simulink library "aeroutilslib"  (Simulink 6.6)
undefined symbols (not defined in the file or in its folder): DiscIntNeverNeededParam, POS_hi, POS_lo, Timestep
libraries: simulink x13, aeroutilslib x1
settings Model: Creator=cox  LastModifiedBy=la1032aw  ExtModeAutoUpdateStatusClock=off

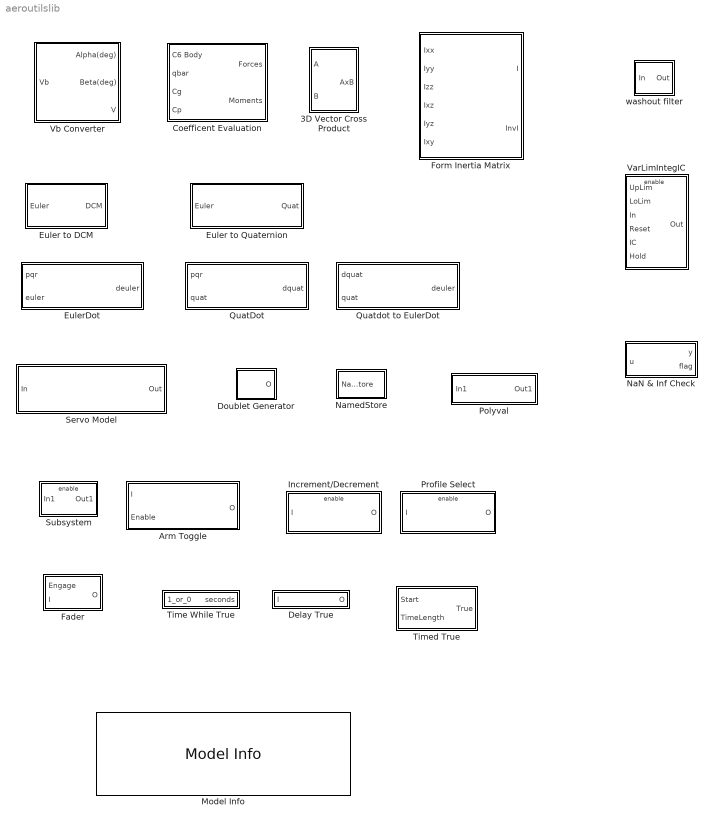
== system aeroutilslib ==
  3D Vector Cross Product : Subsystem
  Arm Toggle : Subsystem
  Coefficent Evaluation : Subsystem  mask{b=1, cbar=1, Sref=1}
      mask prompts: b "Reference Span (b)"; cbar "Reference Chord (cbar)"; Sref "Reference Area (Sref)"
      mask help:
      | Calulates the Force and Moments due to aerodynamic loads from vector of body axes aerodynamic coefficients:
      |    C6body = [Cx Cy Cz Cl Cm Cn].
      | Also requires dynamic pressure, cg/cp locations and reference lengths/area.
  Delay True : Subsystem  mask{holdoff=0, timestep=Timestep}
      mask help: Delays output of "True" value for given time. Outputs boolean. Uses a 32-bit counter instead of a clock source so the output is discrete.
      mask Display: disp([num2str(holdoff) ' sec'])
  Doublet Generator : Subsystem  mask(DoubletGenerator){timeon=[3 10 17], pulsewidth=[2 2 2], amplitude=[0 0 0]}
      mask prompts: timeon "Time Start"; pulsewidth "Pulse Duration"
      mask help:
      | Doublet Generator.
      | Ouputs doublet of specificed amplitude and duration.
      |
      | If start/duration/amplitude parameters are vectors, then output is multichannel.
      mask Display: plot([.1 .3 .3001 .4 .4001 .5  .5001 .7],[0 0 1 1 -1 -1 0 0])
  Euler to DCM : Subsystem
  Euler to Quaternion : Subsystem
  EulerDot : Stateflow chart
  Fader : Subsystem
  Form Inertia Matrix : Stateflow chart
  Increment/Decrement : Subsystem  mask(Increment/Decrement ){Threshold=9}
      mask help:
      | Input is a discrete toggle: +/-1 increments up/down, zero is no change
      | Set the Threshold where the output should wrap around. (1 is the lower limit)
      | Initial value is 1. Output is uint32.
      mask Display: disp(['Threshold: ' num2str(Threshold)])
  Model Info : simulink/Model-Wide Utilities/Model Info  SystemSampleTime=-1  InitialBlockCM=none  BlockCM=none  Frame=on  DisplayStringWithTags=|  HorizontalTextAlignment=Center  LeftAlignmentValue=0.5  SourceBlockDiagram=aeroutilslib  TagMaxNumber=20
      | Aero Utility Library
      | %<ModelVersion>
      | Las modified by %<LastModifiedBy> on %<LastModificationDate>
  NaN & Inf Check : Stateflow chart
  NamedStore : Subsystem  StopFcn=|  mask(Custom To Workspace Block){Npts=inf, VarName=sout, expand=off}
      | %                                                                                       
      | % script: namedstore_stopfcn                                                            
      | %                                                                                       
      | % Workspace script called by NamedStore block as StopFcn callback.                      
      | %                                                                                       
      | % This converts from fixed name array and  variable list                                
      | % into user names structure.   It also optionally expands fields of the                 
      | % structure  into individual variables.                                                 
      |                                                                                         
      | VarName=get_param(gcb,'VarName');                                                       
      |                                                                                         
      |                                                                                         
      | % If data exists                                                                        
      | if exist(strcat(VarName,'_mat'),'var');                                                 
      |   % Grab field names from diagram                                                       
      |    signal_names=get_param(sprintf('%s/Names',gcb),'InputSignals');                      
      |                                                                                         
      |   % Only works for scalar signals...                                                    
      |   % Doing vectors would require pre-compile of diagram,                                 
      |   % and parsing of "CompliedPortDimensions" parameter.                                  
      |   if length(signal_names) ~=  eval(sprintf('size(%s_mat,2)',VarName));                  
      |     fprintf(1,'Structure ''%s'' not formed, namedsore data remains in matrix form\n',...
      |             VarName);                                                                   
      |     error('NamedStore input contains non-scalar signals');                              
      |   end                                                                                   
      |                                                                                         
      |   % Don't want to augment existing variable                                             
      |   eval(sprintf('clear %s',VarName));                                                    
      |                                                                                         
      |   % Loop through each named variable, assign in structure;                              
      |   for cnt=[1:length(signal_names)],                                                     
      |     eval(sprintf('%s.(signal_names{cnt})=%s_mat(:,cnt);',...                            
      |                  VarName,VarName));                                                     
      |   end                                                                                   
      |                                                                                         
      |                                                                                         
      |                                                                                         
      |   % If selected, expand all fields.                                                     
      |   if (strcmp(get_param(gcb,'expand'),'on' ))                                            
      |     eval(sprintf('expand(%s);',VarName));                                               
      |   end                                                                                   
      |  % Delete tmp name variables from workspace                                             
      |   eval(sprintf('clear %s_mat',VarName));                                                
      |   clear cnt VarName signal_names                                                        
      |  end
      mask prompts: Npts "Limit data points to last"; VarName "Variable Name"; expand "Expand Variables in Base Workspace"
      mask help:
      | Saves simulation data to a workspace variable in a structure format.
      | Input is limited to uniquely named scalar signals.
      | Relies on a stop-fcn callback.
      mask init:
      | set_param(sprintf('%s/To Workspace',gcb),'MaxDataPoints',sprintf('%d',Npts));
      | InSig=get_param(sprintf('%s/Names',gcb),'InputSignals');
      | set_param(sprintf('%s/Names',gcb),'OutputSignals',InSig{1});  % Gotta have one..
      | set_param(sprintf('%s/To Workspace',gcb),'VariableName',strcat(VarName,'_mat'));
      | 
      | 
      | 
      | % Check for duplicates, error out
      | [uni,ndx]=unique(InSig);
      | if length(uni)~=length(InSig),
      |  dups=InSig(setdiff([1:length(InSig)],ndx));
      |  dups
      |  error(sprintf('\nDuplicate signal names in named_store block: %s',dups{:}));
      | end
      mask Display: port_label('input',1,VarName);
  Polyval : Subsystem  mask{p=[2 1]}
      mask prompts: p "Polynomial"
      mask help:
      | Embedded MATLAB version of the polyval block.
      | Input polynomial coefficients as a vector in descending order.
      mask Display:
      | disp('y = P(u)\n')
      | disp(['\nO(P) = ' num2str(length(p)-1)])
  Profile Select : Subsystem  mask(Select profile){Profiles=9}
      mask help: Analog input should be normalized between 0 and +1. Block outputs a round number between 1 and the max number of profiles. Output is uint32.
      mask Display: disp(['Profiles: ' num2str(Profiles)])
  QuatDot : Stateflow chart
  Quatdot to EulerDot : Stateflow chart
  Servo Model : Subsystem  mask(Rate and Position Limited Servo){freq=10, RL=999.0, POS_hi=20.0, POS_lo=-30.0}
      mask prompts: freq "Bandwidth, Hz"; RL "Rate Limit:"; POS_hi "Position Limit High:"; POS_lo "Position Limit Low:"
      mask help: First order transfer function: w/(s+w), with rate and position limits.
      mask Help:
      | This block models a first order servo with the initial condition
      | on the integrator set to the steady state value for constant input.
      | The servo is rate and position limited and those values are set
      | in the block parameters.
      mask Display:
      | text(.48,.55,sprintf('%3.1f Hz\nBW',freq),'horizontalAlignment','center');
      | 
      | text(0.18,0.45,sprintf('|d/dt|\n<%0.1f',RL),'horizontalAlignment','center');
      | 
      | text(0.88,0.85,num2str(POS_hi),'horizontalAlignment', 'center');
      | text(0.88,0.2,num2str(POS_lo),'horizontalAlignment', 'center');
      | text(0.73,0.5,'P\nL');
      | 
      | 
      | plot([0.83 0.87 0.93 0.97],[0.4 0.4 0.6 0.6]);
      | plot([0.81 0.99],[0.5 0.5]);
      | plot([0.9 0.9],[0.3 0.7]);
      | plot([0.81 0.99 0.99 0.81 0.81],[0.3 0.3 0.7 0.7 0.3]);
  Subsystem : Subsystem
      mask Type: Toggle Switch
      mask Description: Boolean output toggles between 0 and 1 when an increase is detected in the input
      mask Display: disp('Toggle')
  Time While True : Subsystem  mask{timestep=Timestep}
      mask help: uses a 32-bit and the Timestep variable to output Time While the input signal is true. Output signal is discrete.
  Timed True : Subsystem  mask{timestep=Timestep}
      mask help: Uses a 32-bit counter and the Timestep variable to output a variable time length true signal. Output signal is discrete.
  VarLimIntegIC : Subsystem
  Vb Converter : Subsystem
  washout filter : Subsystem  mask(first order filter){A=1, B=1, C=1}
      mask help:
      | __As__
      |  Bs+C
      |
      | Washout filter  transfer function
      | with integrator IC = input* A/C  at time=0
      mask Help:
      | This block models a washout filter with the initial condition
      | on the integrator set to the steady state value for constant input.
      | A, B and C values are the filter coefficients
      | As / (Bs+C)
      mask Display: dpoly([A 0],[B C]);

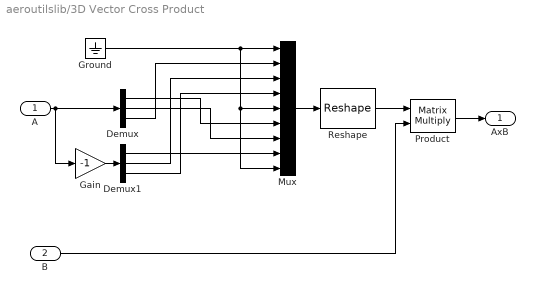
== system aeroutilslib/3D Vector Cross Product ==
  A : Inport
  B : Inport  Port=2
  Demux : Demux  Outputs=3
  Demux1 : Demux  Outputs=3
  Gain : Gain  Gain=-1  SaturateOnIntegerOverflow=on
  Ground : Ground
  Mux : Mux  Inputs=9
  Product : Product  Multiplication=Matrix(*)  SaturateOnIntegerOverflow=on
  Reshape : Reshape  OutputDimensionality=Customize  OutputDimensions=[3,3]
  AxB : Outport
  wires:
  A/1 -> Demux/1, Gain/1
  Product/1 -> AxB/1
  Ground/1 -> Mux/1, Mux/5, Mux/9
  Gain/1 -> Demux1/1
  Demux/3 -> Mux/2
  Demux1/2 -> Mux/3
  Demux1/3 -> Mux/4
  Demux/1 -> Mux/6
  Demux/2 -> Mux/7
  Demux1/1 -> Mux/8
  Mux/1 -> Reshape/1
  Reshape/1 -> Product/1
  B/1 -> Product/2

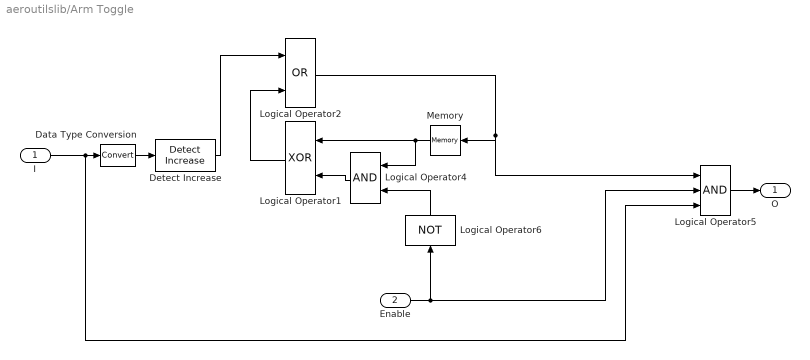
== system aeroutilslib/Arm Toggle ==
  I : Inport
  Enable : Inport  Port=2
  Data Type Conversion : DataTypeConversion  OutDataTypeMode=double
  Detect Increase : simulink/Logic and Bit Operations/Detect Increase  SystemSampleTime=-1  vinit=0.0
  Logical Operator1 : Logic  Orientation=left  Operator=XOR  AllPortsSameDT=off  OutDataTypeMode=Boolean
  Logical Operator2 : Logic  Operator=OR  AllPortsSameDT=off  OutDataTypeMode=Boolean
  Logical Operator4 : Logic  Orientation=left  AllPortsSameDT=off  OutDataTypeMode=Boolean
  Logical Operator5 : Logic  Inputs=3  AllPortsSameDT=off  OutDataTypeMode=Boolean
  Logical Operator6 : Logic  Orientation=up  Operator=NOT  Inputs=3  AllPortsSameDT=off  OutDataTypeMode=Boolean
  Memory : Memory  Orientation=left
  O : Outport
  wires:
  Enable/1 -> Logical Operator6/1, Logical Operator5/2
  Logical Operator2/1 -> Memory/1, Logical Operator5/1
  I/1 -> Logical Operator5/3, Data Type Conversion/1
  Memory/1 -> Logical Operator1/1, Logical Operator4/1
  Logical Operator1/1 -> Logical Operator2/2
  Logical Operator4/1 -> Logical Operator1/2
  Detect Increase/1 -> Logical Operator2/1
  Logical Operator6/1 -> Logical Operator4/2
  Logical Operator5/1 -> O/1
  Data Type Conversion/1 -> Detect Increase/1

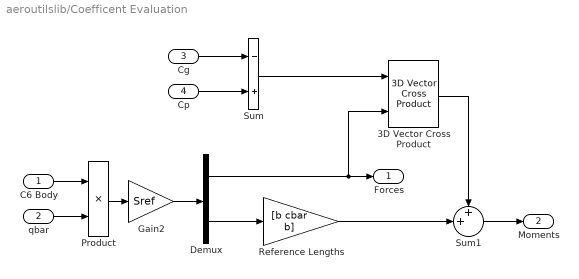
== system aeroutilslib/Coefficent Evaluation ==
  C6 Body : Inport
  qbar : Inport  Port=2
  Cg : Inport  Port=3
  Cp : Inport  Port=4
  3D Vector Cross Product : aeroutilslib/3D Vector Cross Product  SystemSampleTime=-1
  Demux : Demux  Outputs=[3 3]
  Gain2 : Gain  Gain=Sref  SaturateOnIntegerOverflow=on
  Product : Product  SaturateOnIntegerOverflow=on  InputSameDT=on
  Reference Lengths : Gain  Gain=[b cbar b]  SaturateOnIntegerOverflow=on
  Sum : Sum  Inputs=-+  SaturateOnIntegerOverflow=on
  Sum1 : Sum  Inputs=++|  SaturateOnIntegerOverflow=on
  Forces : Outport
  Moments : Outport  Port=2
  wires:
  3D Vector Cross Product/1 -> Sum1/1
  Sum1/1 -> Moments/1
  Reference Lengths/1 -> Sum1/2
  Demux/1 -> Forces/1, 3D Vector Cross Product/2
  Demux/2 -> Reference Lengths/1
  Gain2/1 -> Demux/1
  Product/1 -> Gain2/1
  qbar/1 -> Product/2
  C6 Body/1 -> Product/1
  Cp/1 -> Sum/2
  Cg/1 -> Sum/1
  Sum/1 -> 3D Vector Cross Product/1

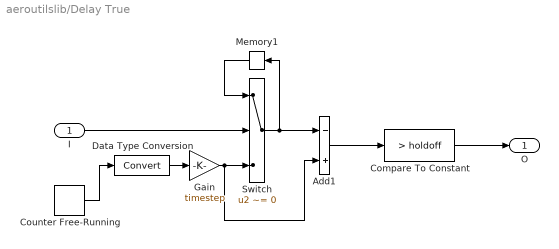
== system aeroutilslib/Delay True ==
  I : Inport
  Add1 : Sum  Inputs=-+  OutScaling=2^-10
  Compare To Constant : simulink/Logic and Bit Operations/Compare To Constant  SystemSampleTime=-1  relop=>  const=holdoff  LogicOutDataTypeMode=boolean  ZeroCross=off
  Counter Free-Running : simulink/Sources/Counter Free-Running  SystemSampleTime=-1  NumBits=32  tsamp=-1
  Data Type Conversion : DataTypeConversion  OutDataTypeMode=double
  Gain : Gain  Gain=timestep
  Memory1 : Memory  Orientation=left
  Switch : Switch  Criteria=u2 ~= 0
  O : Outport
  wires:
  Gain/1 -> Switch/3, Add1/2
  Data Type Conversion/1 -> Gain/1
  Counter Free-Running/1 -> Data Type Conversion/1
  Memory1/1 -> Switch/1
  Switch/1 -> Add1/1, Memory1/1
  I/1 -> Switch/2
  Add1/1 -> Compare To Constant/1
  Compare To Constant/1 -> O/1

== system aeroutilslib/Doublet Generator ==
  Add : Sum  Inputs=+++  OutScaling=2^-10
  DownStep : Step  Time=timeon+pulsewidth  After=-2  SampleTime=0
  Gain : Gain  Gain=amplitude
  UnStep : Step  Time=timeon+2*pulsewidth  SampleTime=0
  UpStep : Step  Time=timeon  SampleTime=0
  O : Outport
  wires:
  UpStep/1 -> Add/1
  DownStep/1 -> Add/2
  UnStep/1 -> Add/3
  Add/1 -> Gain/1
  Gain/1 -> O/1

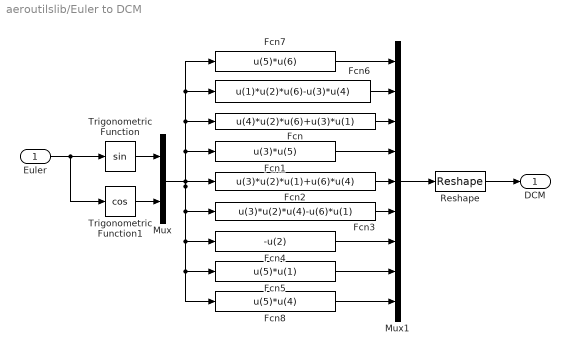
== system aeroutilslib/Euler to DCM ==
  "Euler " : Inport
  Fcn : Fcn  Expr=u(4)*u(2)*u(6)+u(3)*u(1)
  Fcn1 : Fcn  Expr=u(3)*u(5)
  Fcn2 : Fcn  Expr=u(3)*u(2)*u(1)+u(6)*u(4)
  Fcn3 : Fcn  Expr=u(3)*u(2)*u(4)-u(6)*u(1)
  Fcn4 : Fcn  Expr=-u(2)
  Fcn5 : Fcn  Expr=u(5)*u(1)
  Fcn6 : Fcn  Expr=u(1)*u(2)*u(6)-u(3)*u(4)
  Fcn7 : Fcn  Expr=u(5)*u(6)
  Fcn8 : Fcn  Expr=u(5)*u(4)
  Mux : Mux  Inputs=2
  Mux1 : Mux  Inputs=9
  Reshape : Reshape  OutputDimensionality=Customize  OutputDimensions=[3,3]
  Trigonometric Function : Trigonometry
  Trigonometric Function1 : Trigonometry  Operator=cos
  DCM : Outport
  wires:
  "Euler "/1 -> Trigonometric Function1/1, Trigonometric Function/1
  Trigonometric Function/1 -> Mux/1
  Trigonometric Function1/1 -> Mux/2
  Mux/1 -> Fcn/1, Fcn7/1, Fcn6/1, Fcn1/1, Fcn2/1, Fcn4/1, Fcn8/1, Fcn5/1, Fcn3/1
  Mux1/1 -> Reshape/1
  Fcn7/1 -> Mux1/1
  Fcn6/1 -> Mux1/2
  Fcn/1 -> Mux1/3
  Fcn1/1 -> Mux1/4
  Fcn2/1 -> Mux1/5
  Fcn3/1 -> Mux1/6
  Fcn4/1 -> Mux1/7
  Fcn5/1 -> Mux1/8
  Fcn8/1 -> Mux1/9
  Reshape/1 -> DCM/1

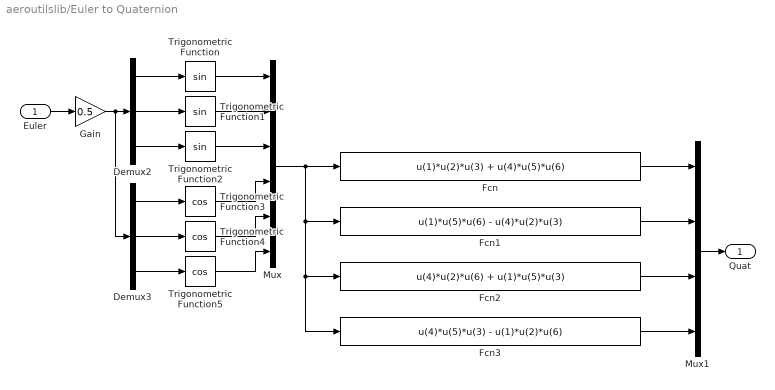
== system aeroutilslib/Euler to Quaternion ==
  Euler : Inport
  Demux2 : Demux  Outputs=3
  Demux3 : Demux  Outputs=3
  Fcn : Fcn  Expr=u(1)*u(2)*u(3) + u(4)*u(5)*u(6)
  Fcn1 : Fcn  Expr=u(1)*u(5)*u(6) - u(4)*u(2)*u(3)
  Fcn2 : Fcn  Expr=u(4)*u(2)*u(6) + u(1)*u(5)*u(3)
  Fcn3 : Fcn  Expr=u(4)*u(5)*u(3) - u(1)*u(2)*u(6)
  Gain : Gain  Gain=0.5
  Mux : Mux  Inputs=6
  Mux1 : Mux
  Trigonometric Function : Trigonometry
  Trigonometric Function1 : Trigonometry
  Trigonometric Function2 : Trigonometry
  Trigonometric Function3 : Trigonometry  Operator=cos
  Trigonometric Function4 : Trigonometry  Operator=cos
  Trigonometric Function5 : Trigonometry  Operator=cos
  Quat : Outport
  wires:
  Gain/1 -> Demux2/1, Demux3/1
  Demux2/1 -> Trigonometric Function/1
  Demux2/2 -> Trigonometric Function1/1
  Demux2/3 -> Trigonometric Function2/1
  Demux3/1 -> Trigonometric Function3/1
  Demux3/2 -> Trigonometric Function4/1
  Demux3/3 -> Trigonometric Function5/1
  Trigonometric Function/1 -> Mux/1
  Trigonometric Function1/1 -> Mux/2
  Trigonometric Function2/1 -> Mux/3
  Trigonometric Function3/1 -> Mux/4
  Trigonometric Function4/1 -> Mux/5
  Trigonometric Function5/1 -> Mux/6
  Mux/1 -> Fcn/1, Fcn1/1, Fcn2/1, Fcn3/1
  Fcn/1 -> Mux1/1
  Fcn1/1 -> Mux1/2
  Fcn2/1 -> Mux1/3
  Fcn3/1 -> Mux1/4
  Euler/1 -> Gain/1
  Mux1/1 -> Quat/1

== system aeroutilslib/Fader ==
  Engage : Inport
  I : Inport  Port=2
  Data Type Conversion : DataTypeConversion  OutDataTypeMode=double
  Divide1 : Product  Inputs=**  OutScaling=2^-10
  Enabled Subsystem : Subsystem  TreatAsAtomicUnit=on
  Rate Limiter +/- 1 sec : RateLimiter  SampleTimeMode=inherited
  O : Outport
  wires:
  Engage/1 -> Data Type Conversion/1, Enabled Subsystem/Enable
  Rate Limiter +/- 1 sec/1 -> Divide1/1
  Divide1/1 -> O/1
  Data Type Conversion/1 -> Rate Limiter +/- 1 sec/1
  I/1 -> Enabled Subsystem/1(I)
  Enabled Subsystem/1(O) -> Divide1/2

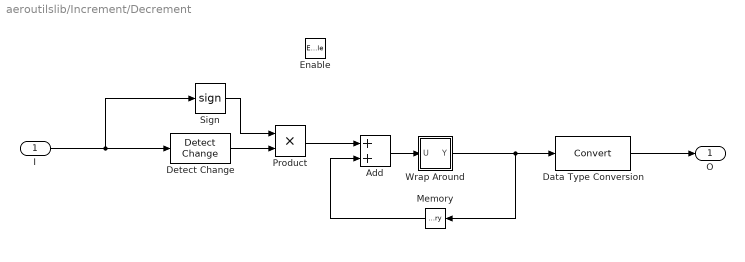
== system aeroutilslib/Increment/Decrement ==
  I : Inport
  Enable : EnablePort
  Add : Sum  OutScaling=2^-10
  Data Type Conversion : DataTypeConversion  OutDataTypeMode=uint32
  Detect Change : simulink/Logic and Bit Operations/Detect Change  SystemSampleTime=-1  vinit=0
  Memory : Memory  Orientation=left
  Product : Product  RndMeth=Zero
  Sign : Signum
  Wrap Around : Subsystem
  O : Outport  InitialOutput=1
  wires:
  Add/1 -> Wrap Around/1(U)
  Memory/1 -> Add/2
  Wrap Around/1(Y) -> Memory/1, Data Type Conversion/1
  Sign/1 -> Product/1
  Detect Change/1 -> Product/2
  Product/1 -> Add/1
  I/1 -> Detect Change/1, Sign/1
  Data Type Conversion/1 -> O/1

== system aeroutilslib/NamedStore ==
  Named Store : Inport
  Bus to Vector : BusToVector
  Names : BusSelector  OutputSignals=eas
  Terminator : Terminator
  To Workspace : ToWorkspace  VariableName=sout_mat  SampleTime=-1  SaveFormat=Array
      settings: MaxDataPoints=Inf
  wires:
  Named Store/1 -> Names/1, Bus to Vector/1
  Names/1 -> Terminator/1  "<eas>"
  Bus to Vector/1 -> To Workspace/1

== system aeroutilslib/Polyval ==
  In1 : Inport
  Embedded MATLAB Function : Stateflow chart
  Out1 : Outport
  wires:
  In1/1 -> Embedded MATLAB Function/1(u)
  Embedded MATLAB Function/1(y) -> Out1/1

== system aeroutilslib/Profile Select ==
  I : Inport
  Enable : EnablePort
  Data Type Conversion : DataTypeConversion  OutDataTypeMode=uint32
  Gain : Gain  Gain=Profiles
  Rounding Function : Rounding  Operator=round
  Saturation : Saturate  UpperLimit=Profiles  LowerLimit=1
  O : Outport  PortDimensions=1  InitialOutput=1
  wires:
  Rounding Function/1 -> Saturation/1
  I/1 -> Gain/1
  Gain/1 -> Rounding Function/1
  Saturation/1 -> Data Type Conversion/1
  Data Type Conversion/1 -> O/1

== system aeroutilslib/Servo Model ==
  In : Inport
  Gain : Gain  Gain=2*pi*freq  SaturateOnIntegerOverflow=on
  Integrator : Integrator  InitialConditionSource=external  LimitOutput=on  UpperSaturationLimit=POS_hi  LowerSaturationLimit=POS_lo  IgnoreLimit=on
  Rate Limiter : Saturate  UpperLimit=RL  LowerLimit=-RL
  Sum : Sum  Inputs=-+|  SaturateOnIntegerOverflow=on  InputSameDT=on
  Out : Outport  PortDimensions=1
  wires:
  In/1 -> Sum/2, Integrator/2
  Rate Limiter/1 -> Integrator/1  "Ydot_lim"
  Integrator/1 -> Out/1, Sum/1  "Y"
  Sum/1 -> Gain/1  "Error"
  Gain/1 -> Rate Limiter/1  "Ydot"

== system aeroutilslib/Subsystem ==
  In1 : Inport
  Enable : EnablePort  StatesWhenEnabling=reset
  Data Type Conversion : DataTypeConversion  OutDataTypeMode=double
  Detect Increase : simulink/Logic and Bit Operations/Detect Increase  SystemSampleTime=-1  vinit=0.0
  Logical Operator : Logic  Operator=XOR  AllPortsSameDT=off  OutDataTypeMode=Boolean
  Memory : Memory  Orientation=left
  Out1 : Outport  OutputWhenDisabled=reset  InitialOutput=0
  wires:
  Memory/1 -> Logical Operator/2
  Logical Operator/1 -> Memory/1, Out1/1
  Detect Increase/1 -> Logical Operator/1
  In1/1 -> Data Type Conversion/1
  Data Type Conversion/1 -> Detect Increase/1

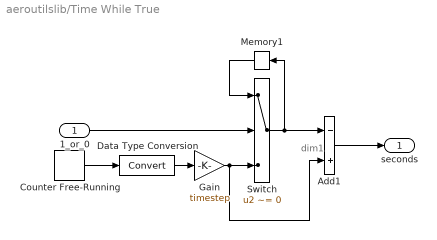
== system aeroutilslib/Time While True ==
  note: dim1
  1_or_0 : Inport
  Add1 : Sum  Inputs=-+  OutScaling=2^-10
  Counter Free-Running : simulink/Sources/Counter Free-Running  SystemSampleTime=-1  NumBits=32  tsamp=-1
  Data Type Conversion : DataTypeConversion  OutDataTypeMode=double
  Gain : Gain  Gain=timestep
  Memory1 : Memory  Orientation=left
  Switch : Switch  Criteria=u2 ~= 0
  seconds : Outport  PortDimensions=1
  wires:
  Gain/1 -> Switch/3, Add1/2
  Data Type Conversion/1 -> Gain/1
  Counter Free-Running/1 -> Data Type Conversion/1
  Memory1/1 -> Switch/1
  Switch/1 -> Add1/1, Memory1/1
  1_or_0/1 -> Switch/2
  Add1/1 -> seconds/1

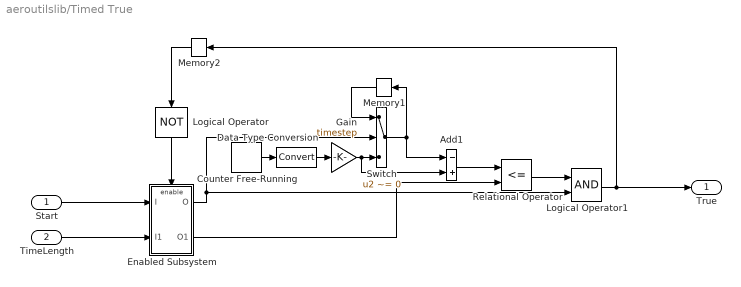
== system aeroutilslib/Timed True ==
  Start : Inport
  TimeLength : Inport  Port=2
  Add1 : Sum  Inputs=-+  OutScaling=2^-10
  Counter Free-Running : simulink/Sources/Counter Free-Running  SystemSampleTime=-1  NumBits=32  tsamp=-1
  Data Type Conversion : DataTypeConversion  OutDataTypeMode=double
  Enabled Subsystem : Subsystem  TreatAsAtomicUnit=on
  Gain : Gain  Gain=timestep
  Logical Operator : Logic  Orientation=down  Operator=NOT  AllPortsSameDT=off  OutDataTypeMode=Boolean
  Logical Operator1 : Logic  AllPortsSameDT=off  OutDataTypeMode=Boolean
  Memory1 : Memory  Orientation=left
  Memory2 : Memory  Orientation=left
  Relational Operator : RelationalOperator  Operator=<=  LogicOutDataTypeMode=Boolean
  Switch : Switch  Criteria=u2 ~= 0
  True : Outport
  wires:
  Logical Operator1/1 -> True/1, Memory2/1
  Relational Operator/1 -> Logical Operator1/1
  Add1/1 -> Relational Operator/1
  Enabled Subsystem/1(O) -> Switch/2, Logical Operator1/2
  Switch/1 -> Memory1/1, Add1/1
  Memory1/1 -> Switch/1
  TimeLength/1 -> Enabled Subsystem/2(I1)
  Start/1 -> Enabled Subsystem/1(I)
  Enabled Subsystem/2(O1) -> Relational Operator/2
  Memory2/1 -> Logical Operator/1
  Logical Operator/1 -> Enabled Subsystem/Enable
  Data Type Conversion/1 -> Gain/1
  Counter Free-Running/1 -> Data Type Conversion/1
  Gain/1 -> Add1/2, Switch/3

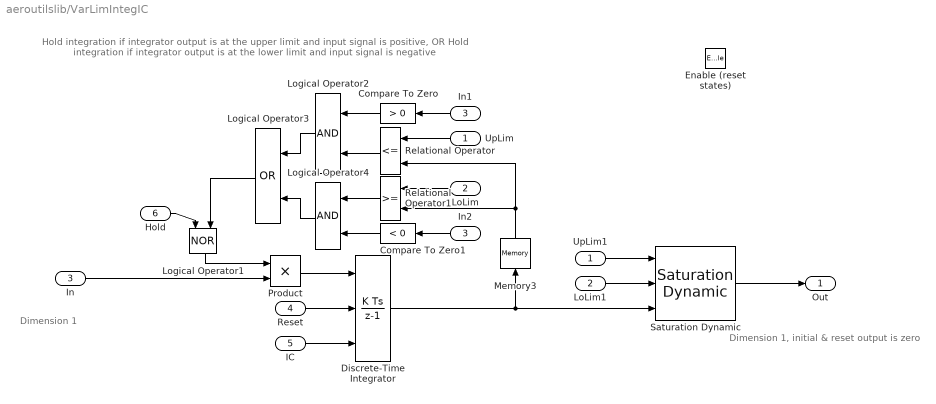
== system aeroutilslib/VarLimIntegIC ==
  note: Dimension 1
  note: Dimension 1,
      | initial & reset output is zero
  note: Hold integration if integrator output is at the upper limit and input signal is positive, OR
      | Hold integration if integrator output is at the lower limit and input signal is negative
  UpLim : Inport  Orientation=left
  LoLim : Inport  Orientation=left  Port=2
  In : Inport  Port=3  PortDimensions=1
  Reset : Inport  Port=4
  IC : Inport  Port=5
  Hold : Inport  Port=6
  Enable (reset states) : EnablePort  StatesWhenEnabling=reset
  Compare To Zero : simulink/Logic and Bit Operations/Compare To Zero  Orientation=left  SystemSampleTime=-1  relop=>  LogicOutDataTypeMode=boolean  ZeroCross=off
  Compare To Zero1 : simulink/Logic and Bit Operations/Compare To Zero  Orientation=left  SystemSampleTime=-1  relop=<  LogicOutDataTypeMode=boolean  ZeroCross=off
  Discrete-Time Integrator : DiscreteIntegrator  ExternalReset=level  InitialConditionSource=external  SampleTime=Timestep  ICPrevOutput=DiscIntNeverNeededParam  ICPrevScaledInput=DiscIntNeverNeededParam
  In1 : InportShadow  Orientation=left  Port=3  PortDimensions=1  LatchByCopyingInsideSignal=off
  In2 : InportShadow  Orientation=left  Port=3  PortDimensions=1  LatchByCopyingInsideSignal=off
  LoLim1 : InportShadow  Port=2  LatchByCopyingInsideSignal=off
  Logical Operator1 : Logic  Orientation=down  Operator=NOR  AllPortsSameDT=off  OutDataTypeMode=Specify via dialog  LogicDataType=float('double')
  Logical Operator2 : Logic  Orientation=left  AllPortsSameDT=off  OutDataTypeMode=Specify via dialog  LogicDataType=float('double')
  Logical Operator3 : Logic  Orientation=left  Operator=OR  AllPortsSameDT=off  OutDataTypeMode=Boolean
  Logical Operator4 : Logic  Orientation=left  AllPortsSameDT=off  OutDataTypeMode=Specify via dialog  LogicDataType=float('double')
  Memory3 : Memory  Orientation=up
  Product : Product  RndMeth=Zero
  Relational Operator : RelationalOperator  Orientation=left  Operator=<=  LogicOutDataTypeMode=Boolean
  Relational Operator1 : RelationalOperator  Orientation=left  LogicOutDataTypeMode=Boolean
  Saturation Dynamic : simulink/Discontinuities/Saturation Dynamic  SystemSampleTime=-1
  UpLim1 : InportShadow  Port=1  LatchByCopyingInsideSignal=off
  Out : Outport  PortDimensions=1  OutputWhenDisabled=reset  InitialOutput=0
  wires:
  Logical Operator1/1 -> Product/1
  Product/1 -> Discrete-Time Integrator/1
  In/1 -> Product/2
  Discrete-Time Integrator/1 -> Memory3/1, Saturation Dynamic/3
  IC/1 -> Discrete-Time Integrator/3
  LoLim/1 -> Relational Operator1/1
  UpLim/1 -> Relational Operator/1
  Reset/1 -> Discrete-Time Integrator/2
  Relational Operator1/1 -> Logical Operator4/1
  Saturation Dynamic/1 -> Out/1
  UpLim1/1 -> Saturation Dynamic/1
  LoLim1/1 -> Saturation Dynamic/2
  Hold/1 -> Logical Operator1/1
  Memory3/1 -> Relational Operator1/2, Relational Operator/2
  In1/1 -> Compare To Zero/1
  Compare To Zero/1 -> Logical Operator2/1
  Relational Operator/1 -> Logical Operator2/2
  In2/1 -> Compare To Zero1/1
  Compare To Zero1/1 -> Logical Operator4/2
  Logical Operator2/1 -> Logical Operator3/1
  Logical Operator4/1 -> Logical Operator3/2
  Logical Operator3/1 -> Logical Operator1/2

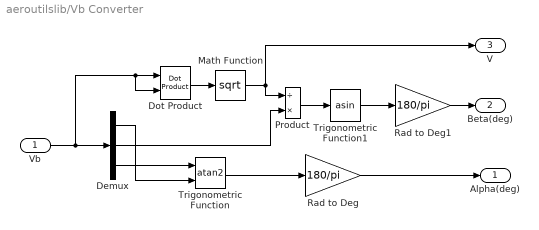
== system aeroutilslib/Vb Converter ==
  Vb : Inport
  Demux : Demux  Outputs=3
  Dot Product : simulink/Math Operations/Dot Product  InputSameDT=on  OutDataType=sfix(16)  OutScaling=2^-10  DoSatur=off
  Math Function : Math  Operator=sqrt  SaturateOnIntegerOverflow=on
  Product : Product  Inputs=/*  SaturateOnIntegerOverflow=on
  Rad to Deg : Gain  Gain=180/pi  SaturateOnIntegerOverflow=on
  Rad to Deg1 : Gain  Gain=180/pi  SaturateOnIntegerOverflow=on
  Trigonometric Function : Trigonometry  Operator=atan2
  Trigonometric Function1 : Trigonometry  Operator=asin
  Alpha(deg) : Outport
  Beta(deg) : Outport  Port=2
  V : Outport  Port=3
  wires:
  Demux/2 -> Product/2
  Math Function/1 -> V/1, Product/1
  Product/1 -> Trigonometric Function1/1
  Demux/3 -> Trigonometric Function/1
  Demux/1 -> Trigonometric Function/2
  Dot Product/1 -> Math Function/1
  Vb/1 -> Demux/1, Dot Product/1, Dot Product/2
  Trigonometric Function/1 -> Rad to Deg/1
  Rad to Deg/1 -> Alpha(deg)/1
  Trigonometric Function1/1 -> Rad to Deg1/1
  Rad to Deg1/1 -> Beta(deg)/1

== system aeroutilslib/washout filter ==
  In : Inport
  Discrete-Time Integrator : DiscreteIntegrator  InitialConditionSource=external  SampleTime=Timestep  UpperSaturationLimit=POS_hi  LowerSaturationLimit=POS_lo  ICPrevOutput=DiscIntNeverNeededParam  ICPrevScaledInput=DiscIntNeverNeededParam
  Gain : Gain  Gain=A/B  SaturateOnIntegerOverflow=on
  Sum : Sum  Inputs=-+|  SaturateOnIntegerOverflow=on  InputSameDT=on
  gain : Gain  Orientation=left  Gain=C/A  SaturateOnIntegerOverflow=on
  gain2 : Gain  Gain=A/C  SaturateOnIntegerOverflow=on
  Out : Outport
  wires:
  gain2/1 -> Discrete-Time Integrator/2
  gain/1 -> Sum/1
  Sum/1 -> Gain/1  "Error"
  In/1 -> gain2/1, Sum/2
  Gain/1 -> Out/1, Discrete-Time Integrator/1  "Ydot"
  Discrete-Time Integrator/1 -> gain/1  "Y"

== system aeroutilslib/Fader/Enabled Subsystem ==
  I : Inport
  Enable : EnablePort
  O : Outport
  wires:
  I/1 -> O/1

== system aeroutilslib/Increment/Decrement/Wrap Around ==
  note: U(k)
  U : Inport
  Constant : Constant
  Constant1 : Constant  Value=Threshold
  Constant2 : Constant  Value=Threshold
  Embedded MATLAB Function : Stateflow chart
  FixPt Data Type Duplicate1 : simulink/Signal Attributes/Data Type Duplicate  NumInputPorts=4
  Multiport Switch : MultiPortSwitch  Inputs=3
  Y : Outport  InitialOutput=0
  wires:
  Constant/1 -> Multiport Switch/3, FixPt Data Type Duplicate1/2
  Constant1/1 -> Multiport Switch/4, FixPt Data Type Duplicate1/3
  Multiport Switch/1 -> Y/1, FixPt Data Type Duplicate1/1
  U/1 -> Embedded MATLAB Function/1(u), FixPt Data Type Duplicate1/4, Multiport Switch/2
  Embedded MATLAB Function/1(y) -> Multiport Switch/1
  Constant2/1 -> Embedded MATLAB Function/2(Threshold)

== system aeroutilslib/Timed True/Enabled Subsystem ==
  I : Inport
  I1 : Inport  Port=2
  Enable : EnablePort
  O : Outport
  O1 : Outport  Port=2
  wires:
  I1/1 -> O1/1
  I/1 -> O/1

== matlab function Form Inertia Matrix ==
  settings: updateMethod=DISCRETE  sampleTime=Timestep
  data: Ixx input double size=1; I output inherited size=[3 3]; Iyy input inherited size=1; Izz input inherited size=1; Ixz input inherited size=1; Iyz input inherited size=1; Ixy input inherited size=1; InvI output inherited size=[3 3]
function [I,InvI] = Inertia(Ixx,Iyy,Izz,Ixz,Iyz,Ixy)
% This block supports an embeddable subset of the MATLAB language.
% See the help menu for details. 

I=[ Ixx, -Ixy, -Ixz;
   -Ixy,  Iyy, -Iyz;
   -Ixz, -Iyz,   Izz ];

det = Ixx*Iyy*Izz-Ixx*Iyz^2-Ixy^2*Izz-2*Ixy*Ixz*Iyz-Ixz^2*Iyy;

adjoint=[...
Iyy*Izz-Iyz^2,    Ixy*Izz+Ixz*Iyz, Ixy*Iyz+Ixz*Iyy;...
Ixy*Izz+Ixz*Iyz,   Ixx*Izz-Ixz^2,  Ixx*Iyz+Ixy*Ixz;...
Ixy*Iyz+Ixz*Iyy,  Ixx*Iyz+Ixy*Ixz,   Ixx*Iyy-Ixy^2     ];

InvI=adjoint/det;

== matlab function Quatdot to EulerDot ==
  settings: updateMethod=DISCRETE  sampleTime=Timestep
  data: dquat input inherited size=4; quat input inherited size=4; deuler output inherited size=3
function deuler = q2de(dquat,quat)
% This block supports an embeddable subset of the MATLAB language.
% See the help menu for details. 

% Quaternion
e0=quat(1);
ex=quat(2);
ey=quat(3);
ez=quat(4);

% Derivative of quaternion
e0d = dquat(1);
exd = dquat(2);
eyd = dquat(3);
ezd = dquat(4);

% Transform d/dt quat into d/dt euler, big chain rule
 theta_dot = -2*(ez*exd + ex*ezd - e0*eyd - ey*e0d)...
             / sqrt(1 - 4*ex*ex*ez*ez + 8*ey*ez*ex*e0 - 4*ey*ey*e0*e0);
 psi_dot   =  2* (      exd*ey*(-ex*ex - ey*ey - ez*ez + e0*e0)...
                            + eyd*ex*( ex*ex + ey*ey - ez*ez + e0*e0)...
                            + ezd*e0*( ex*ex - ey*ey + ez*ez + e0*e0)...
                            + e0d*ez*( ex*ex - ey*ey - ez*ez - e0*e0)...
                            + 2*(ex*ey*ez*ezd - ex*ey*e0*e0d - ez*e0*ex*exd + ez*e0*ey*eyd) )...
                          /...
                           (  ex*ex*(ex*ex + 2*(ey*ey - ez*ez + e0*e0))...
                            + ey*ey*(ey*ey + 2*(ez*ez - e0*e0))...
                            + ez*ez*(ez*ez + 2*e0*e0)...
                            + e0*e0*e0*e0...
                            + 8*ey*ez*ex*e0);
                        
                        
phi_dot   = -2* (      eyd*ez*( ex*ex - ey*ey - ez*ez - e0*e0)...
                            + ezd*ey*( ex*ex + ey*ey + ez*ez - e0*e0)...
                            + exd*e0*(-ex*ex + ey*ey - ez*ez - e0*e0)...
                            + e0d*ex*( ex*ex + ey*ey - ez*ez + e0*e0)...
                            + 2*(-ey*ez*ex*exd + ey*ez*e0*e0d - ex*e0*ey*eyd + ex*e0*ez*ezd) )...
                          /...
                           (  ex*ex*(ex*ex + 2*(ey*ey - ez*ez + e0*e0))...
                            + ey*ey*(ey*ey + 2*(ez*ez - e0*e0))...
                            + ez*ez*(ez*ez + 2*e0*e0)...
                            + e0*e0*e0*e0...
                            + 8*ey*ez*ex*e0);
                        

deuler=[phi_dot; theta_dot; psi_dot];

== matlab function EulerDot ==
  settings: updateMethod=DISCRETE  sampleTime=Timestep
  data: pqr input inherited size=3; deuler output inherited size=3; euler input inherited size=3
function deuler = e2de(pqr,euler)
% This block supports an embeddable subset of the MATLAB language.
% See the help menu for details. 

P=pqr(1);
Q=pqr(2);
R=pqr(3);

phi=euler(1);
theta=euler(2);
psi=euler(3);

c_phi=cos(phi);
s_phi=sin(phi);
c_theta=cos(theta);
s_theta=sin(theta);

phi_dot   = P + (1/c_theta)*(s_phi*s_theta*Q + c_phi*s_theta*R);
theta_dot = c_phi*Q - s_phi*R;
psi_dot   = (1/c_theta)*(s_phi*Q + c_phi*R);

deuler=[phi_dot; theta_dot; psi_dot];

== matlab function Increment/Decrement/Wrap Around/Embedded MATLAB Function ==
  data: u input inherited; y output inherited; Threshold input inherited
function y = fcn(u,Threshold)
% This block supports the Embedded MATLAB subset.
% See the help menu for details. 


if u > Threshold
    y = 2;
elseif u < 1
    y = 3;
else
    y = 1;
end

== matlab function QuatDot ==
  settings: updateMethod=DISCRETE  sampleTime=Timestep
  data: pqr input inherited size=3; dquat output inherited size=4; quat input inherited size=4
function dquat = q2dq(pqr,quat)
% This block supports an embeddable subset of the MATLAB language.
% See the help menu for details. 

P=pqr(1);
Q=pqr(2);
R=pqr(3);

dquat = 0.5 * [ 0 -P -Q -R;
                P  0  R -Q;
                Q -R  0  P;
                R  Q -P  0 ] * quat;

== matlab function Polyval/Embedded MATLAB Function ==
  data: u input inherited; y output inherited; p parameter inherited
function y = fcn(u,p)
% This block supports the Embedded MATLAB subset.
% See the help menu for details. 


y = sum(p.*u.^(length(p)-1:-1:0));

== matlab function NaN & Inf Check ==
  settings: updateMethod=DISCRETE  sampleTime=Timestep
  data: u input inherited; y output inherited; flag output inherited
function [y,flag] = fcn(u)
% Block checks the input u for +/- Infinity and Not a Number. Any Inf or NaN 
% values are replaced with the last valid (non-Inf/NaN) input. Inputs/outputs are 
% vectorized.
%
% Bug: library version of this block must have the same size inputs wherever it is
% used in the model. One library instance of this block exists in the LPS_lib, 
% and two non-library instances of this block exist in Telemetry_lib.
%
% Author: Austin Murch (Austin.M.Murch@nasa.gov)
% Created: 11/12/2008
%

persistent y0

y  = u;

% Initialize persistent variable
if isempty(y0)
    y0 = zeros(size(u));
end

% Find any NaNs or Infs.
indx = isnan(u) | isinf(u);
if any(indx)
    for i = 1:length(indx) % Note: logical indexing is not supported in Embedded MATLAB, hence the for loop
        if indx(i)
            y(i) = y0(i);
        else
            y0(i) = y(i);
        end
    end
    flag = uint8(1);
else
    flag = uint8(0);
    y0 = y;
end
